simulink model "Linear_Kalman_filter"  (R2025a)
settings: Solver=ode4  StartTime=0.0  StopTime=10.0  FixedStep=0.01  RelTol=1e-3
undefined symbols (not defined in the file): Ac, Bc, Cc, L, psi_op, theta_op
settings Model: Creator=bulve  LastModifiedBy=BjørnErikUlveraker

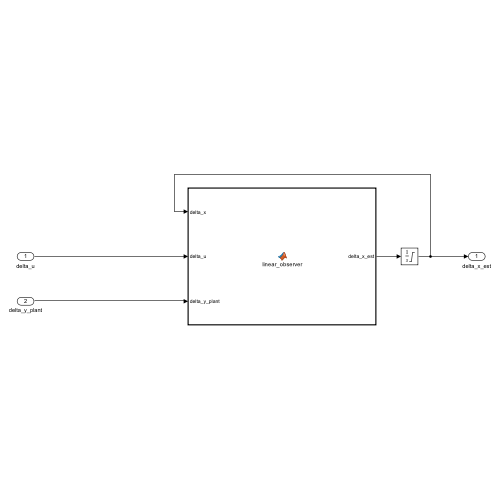
[thumbnail: Simulink's stored preview of the top-level diagram]
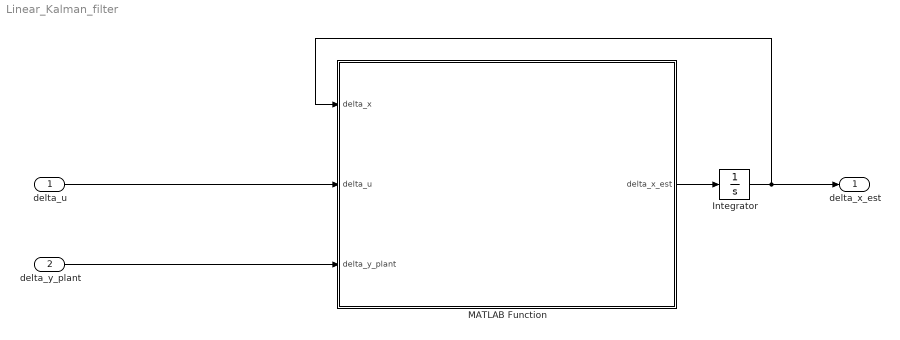
== system Linear_Kalman_filter ==
  delta_u : Inport
  delta_y_plant : Inport  Port=2
  Integrator : Integrator  LimitOutput=on  UpperSaturationLimit=[45*pi/180-theta_op;pi-psi_op;inf;inf]  LowerSaturationLimit=[-45*pi/180-theta_op;0-psi_op;-inf;-inf]
  MATLAB Function : MATLAB Function  TreatAsAtomicUnit=on
  delta_x_est : Outport
  wires:
  MATLAB Function/1(delta_x_est) -> Integrator/1
  delta_y_plant/1 -> MATLAB Function/3(delta_y_plant)
  Integrator/1 -> delta_x_est/1, MATLAB Function/1(delta_x)
  delta_u/1 -> MATLAB Function/2(delta_u)

== matlab function Linear_Kalman_filter/MATLAB Function ==
  data: delta_x input size=[4 1]; delta_x_est output size=[4 1]; delta_u input size=[2 1]; delta_y_plant input size=[2 1]; Ac parameter; Bc parameter; Cc parameter; L parameter
function delta_x_est = linear_observer(delta_x,delta_u,delta_y_plant, Ac, Bc, Cc, L)

delta_x       = delta_x(:);        % 4x1
delta_u       = delta_u(:);        % force column 2x1
delta_y_plant = delta_y_plant(:);  % force column 2x1

y_est = Cc*delta_x;

delta_x_est = Ac*delta_x +Bc*delta_u + L*(delta_y_plant-y_est);
